simulink model "motor"  (R2019b)
settings: Solver=VariableStepAuto  StartTime=0.0  StopTime=10.0  RelTol=1e-3
values from neighbouring files (symbols this model uses):
  L = collect(simplify(2*L_r + L_a + L_b + L_c))    [VAB_non_lineare.m]    (also in fdt_vab_lineare.m; fdt_vab_non_lineare.m = vpa(collect(simplify(2*L_r + L_a + L_b + L_c)),4))
  R = [cos(qz)  -sin(qz) 0;sin(qz) cos(qz) 0; 0 0 1]    [call_plot.m]
undefined symbols (not defined in the file or in its folder): J_m_star, k_t, sigbuilder_block
libraries: cstblocks x1
settings Model: Creator=AndreaCalegari  LastModifiedBy=AndreaCalegari

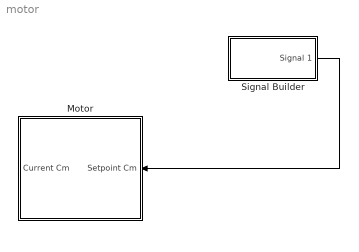
== system motor ==
  "Motor " : Subsystem
  Signal Builder : Subsystem  Tag=STV Subsys  LoadFcn=sigbuilder_block('load');  StartFcn=sigbuilder_block('start');  StopFcn=sigbuilder_block('stop');  ClipboardFcn=sigbuilder_block('clipboard');  mask(Sigbuilder block){tuvar=[0:10]}
      mask help: Simulink:masks:SigbuilderBlock_MD
      mask init:
      | if ~strcmp(get_param(bdroot(gcbh),'SimulationStatus'),'stopped') tuvar = sigbuilder_block('maskInit'); end
      settings: CopyFcn=sigbuilder_block('copy');  DeleteFcn=sigbuilder_block('delete');  ModelCloseFcn=sigbuilder_block('modelClose');  PreSaveFcn=sigbuilder_block('preSave');  PauseFcn=sigbuilder_block('pause');  ContinueFcn=sigbuilder_block('continue');  NameChangeFcn=sigbuilder_block('namechange');  OpenFcn=sigbuilder_block('open',[398.25 57.75 550.5 359.25 ]);  CloseFcn=sigbuilder_block('close');
      mask Display: plot(0, 0, 100, 100,[2, 2, 32, 32, 2], [68, 8, 8, 68, 68],[32, 2], [38, 38], [32, 19, 2],[53, 60, 44], [32, 17, 17, 2],[16, 16, 31, 31]);txt = getActiveGroup(gcbh);text(2, 100, txt,'verticalAlignment', 'top');
  wires:
  Signal Builder/1(Signal 1) -> "Motor "/1(Setpoint Cm)

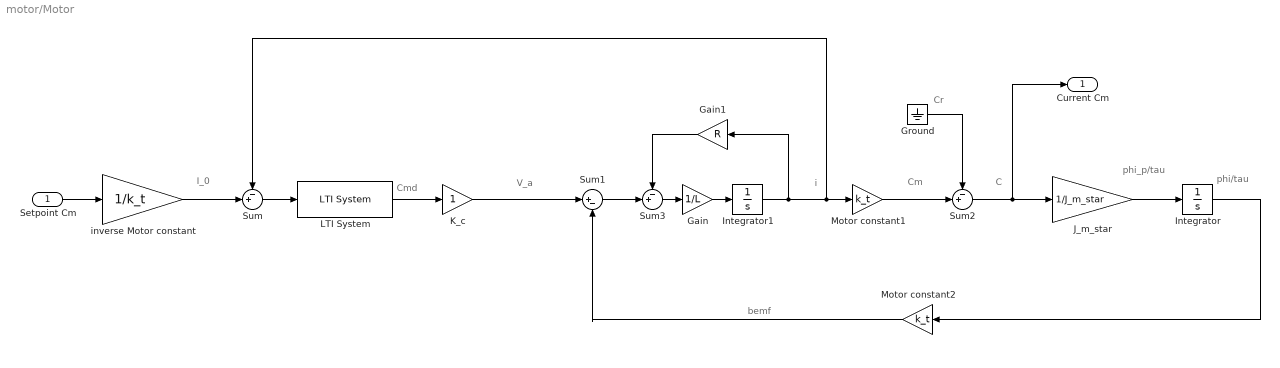
== system motor/Motor  ==
  note: bemf
  note: phi/tau
  note: phi_p/tau
  note: C
  note: i
  note: Cmd
  note: V_a
  note: I_0
  note: Cm
  note: Cr
  Setpoint Cm : Inport
  Gain : Gain  Gain=1/L
  Gain1 : Gain  Gain=R
  Ground : Ground
  Integrator : Integrator
  Integrator1 : Integrator  LimitOutput=on  UpperSaturationLimit=20  LowerSaturationLimit=-20
  "J_m_star " : Gain  Gain=1/J_m_star
  K_c : Gain
  LTI System : cstblocks/LTI System  sys=PI_I  IC=[]
  Motor constant1 : Gain  Gain=k_t
  Motor constant2 : Gain  Gain=k_t
  Sum : Sum  Inputs=-+|
  Sum1 : Sum  Inputs=|+-
  Sum2 : Sum  Inputs=-+|
  Sum3 : Sum  Inputs=-+|
  inverse Motor constant : Gain  Gain=1/k_t
  "Current Cm " : Outport
  wires:
  Integrator/1 -> Motor constant2/1
  Motor constant1/1 -> Sum2/2
  K_c/1 -> Sum1/1
  Integrator1/1 -> Gain1/1, Sum/1, Motor constant1/1
  inverse Motor constant/1 -> Sum/2
  Sum2/1 -> "Current Cm "/1, "J_m_star "/1
  "J_m_star "/1 -> Integrator/1
  Ground/1 -> Sum2/1
  Motor constant2/1 -> Sum1/2
  Setpoint Cm/1 -> inverse Motor constant/1
  Gain/1 -> Integrator1/1
  Sum3/1 -> Gain/1
  Sum1/1 -> Sum3/2
  Gain1/1 -> Sum3/1
  Sum/1 -> LTI System/1
  LTI System/1 -> K_c/1

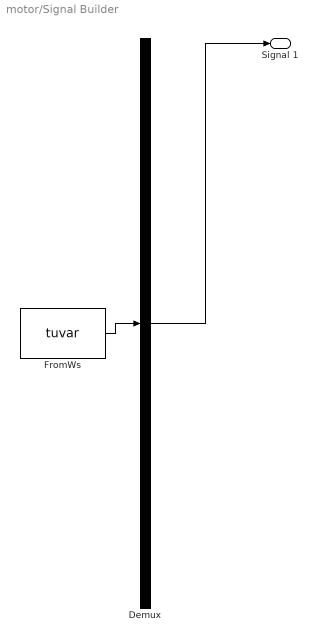
== system motor/Signal Builder ==
  Demux : Demux  Tag=STV Demux  Outputs=1
  FromWs : FromWorkspace  Tag=STV FromWs  VariableName=tuvar  SampleTime=0
      SigBuilderData=|
      | common.afterFinalStr = 'Extrapolate'
      | common.sampleTime = 0
      | dataSet.timeRange = [0 10]
      | dataSet.name = 'Group 1'
      | sbobj.Groups.Name = 'Group 1'
      | sbobj.Groups.Signals.Name = 'Signal 1'
      | sbobj.Groups.Signals.XData = [0 0.01 0.01 0.1 0.1 10]
      | sbobj.Groups.Signals.YData = [28.1 28.1 29.1 29.1 28.1 28.1]
  Signal 1 : Outport  Tag=STV Outport
  wires:
  Demux/1 -> Signal 1/1
  FromWs/1 -> Demux/1
